simulink model "robotSafeTrajectoryTracking"  (R2024a)
settings: Solver=FixedStepAuto  StartTime=0.0  StopTime=20  FixedStep=0.005  RelTol=1e-3
PostLoadFcn:
  | % load sawyer robot mesh for visualization
  | exampleHelperLoadSawyerMesh()
InitFcn:
  | objectPos = 0.6;
  | refPos = 0.185;
StartFcn:
  | objectPos = 0.6;
model workspace (MAT data in the model file):
  p = [0  0.0291358024691  0  -0.0538271604938  0  0.0247111111111  -0.0818790123457; 0  -0.218518518519  0  0.403703703704  0  -0.185333333333  0.614092592593; 0  0.437037037037  0  -0.807407407407  0  0.370666666667  -1.22818518519; 0  0  0  0  0  0  0; 0  0  0  0  0  0  0; 0  -1.18  0  2.18  0  -1.0008  3.3161]
  q0 = [0; -1.18; 0; 2.18; 0; -1.0008; 3.3161]
  q1 = [0; 0; 0; 0; 0; 0; 0]
  sawyer : robotics.RigidBodyTree (value not decoded)
  tDuration = 3
  tStart = 0.5
undefined symbols (not defined in the file or in its folder): X, Y, Z
libraries: sm_lib x153, nesl_utility x33, robotmaniplib x5, robotcorelib x2
(part 1 of 4)
CloseFcn:
  | clear objectPos refPos
settings Model: Creator=The MathWorks, Inc.  LastModifiedBy=amazon
settings SolverCC: AlgebraicLoopSolver=TrustRegion  MinimalZcImpactIntegration=on
settings DataIOCC: ReturnWorkspaceOutputs=off
settings DebuggingCC: UnconnectedInputMsg=warning  UnconnectedOutputMsg=warning  UnconnectedLineMsg=warning  ArithmeticOperatorsInVariantConditions=warning
settings ModelReferenceCC: EnableRefExpFcnMdlSchedulingChecks=on
settings SFSimCC: SimUseLocalCustomCode=off  CustomCodeUndefinedFunction=UseInterfaceOnly
settings RTWCC: RTWUseLocalCustomCode=off  GPUComputeCapability=3.5  DLArmComputeVersion=19.05
settings DiagnosticsConfigSet: SimMechanicsRigidlyBoundBlock=warning

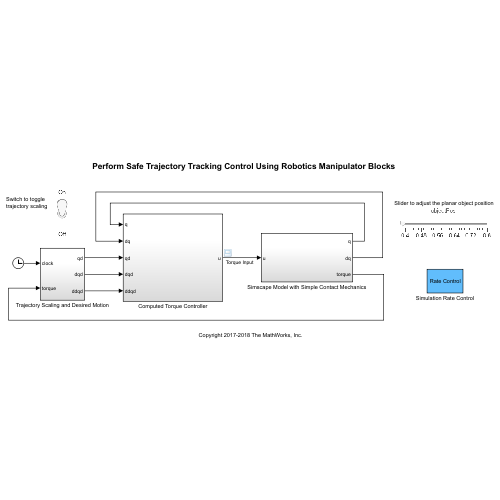
[thumbnail: Simulink's stored preview of the top-level diagram]
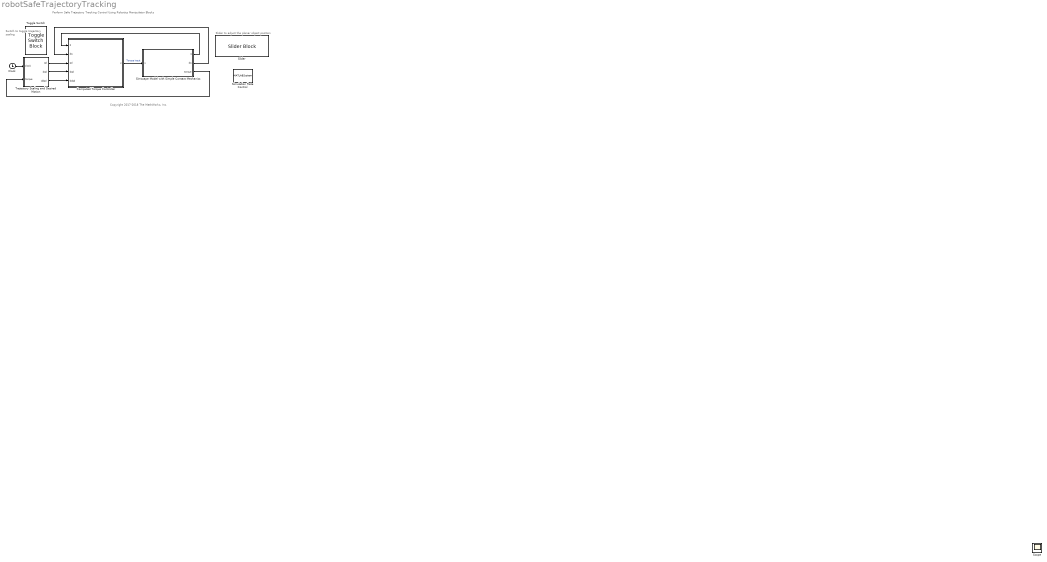
== system robotSafeTrajectoryTracking ==
  note: Perform Safe Trajectory Tracking Control Using Robotics Manipulator Blocks
  note: Switch to toggle
      | trajectory scaling
  note: Copyright 2017-2018 The MathWorks, Inc.
  note: Slider to adjust the planar object position
  Clock : Clock
  Computed Torque Controller : Subsystem
  Simscape Model with Simple Contact Mechanics : Subsystem
  Simulation Rate Control : MATLABSystem  System=ExampleHelperSimulationRateControl  SampleTime=0.005
      mask Type: ExampleHelperSimulationRateControl
      mask Display: disp('Rate Control');
  Slider : SliderBlock  ScaleMin=0.40000000000000002  ScaleMax=0.80000000000000004
  Toggle Switch : ToggleSwitchBlock  LabelPosition=Hide
      settings: Values={{'Off', 'On'}, [0 1]}
  Trajectory Scaling and Desired Motion : Subsystem
  Scope : Scope
  wires:
  Trajectory Scaling and Desired Motion/1(qd) -> Computed Torque Controller/3(qd)
  Trajectory Scaling and Desired Motion/2(dqd) -> Computed Torque Controller/4(dqd)
  Trajectory Scaling and Desired Motion/3(ddqd) -> Computed Torque Controller/5(ddqd)
  Clock/1 -> Trajectory Scaling and Desired Motion/1(clock)
  Simscape Model with Simple Contact Mechanics/1(q) -> Computed Torque Controller/1(q)
  Simscape Model with Simple Contact Mechanics/2(dq) -> Computed Torque Controller/2(dq)
  Simscape Model with Simple Contact Mechanics/3(torque) -> Trajectory Scaling and Desired Motion/2(torque)
  Computed Torque Controller/1(u) -> Simscape Model with Simple Contact Mechanics/1(u)  "Torque Input"

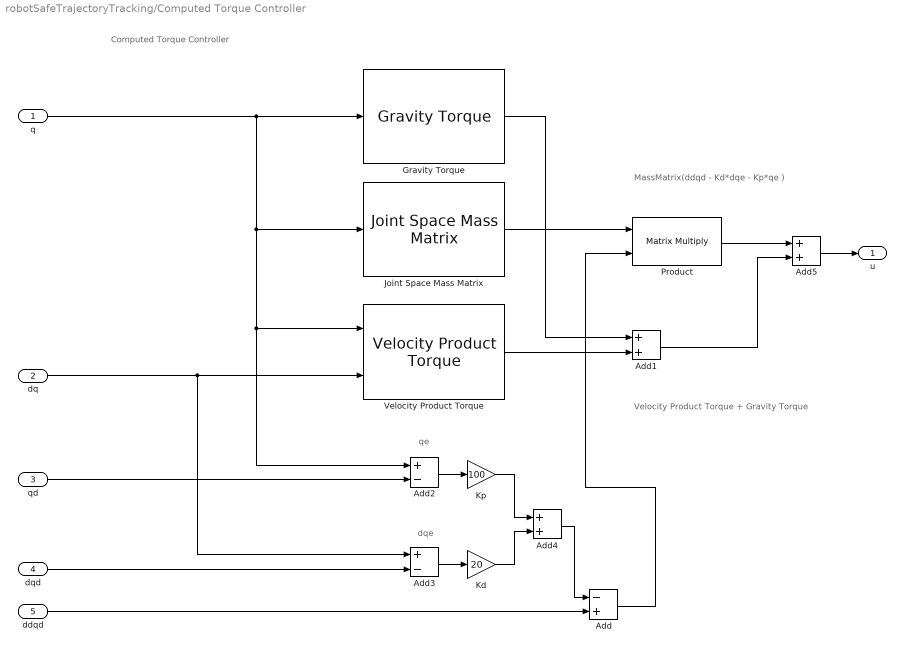
== system robotSafeTrajectoryTracking/Computed Torque Controller ==
  note: qe
  note: dqe
  note: Velocity Product Torque + Gravity Torque
  note: MassMatrix(ddqd - Kd*dqe - Kp*qe )
  note: Computed Torque Controller
  q : Inport
  dq : Inport  Port=2
  qd : Inport  Port=3
  dqd : Inport  Port=4
  ddqd : Inport  Port=5
  Add : Sum  Inputs=-+
  Add1 : Sum
  Add2 : Sum  Inputs=+-
  Add3 : Sum  Inputs=+-
  Add4 : Sum
  Add5 : Sum
  Gravity Torque : robotmaniplib/Gravity Torque  RigidBodyTree=sawyer  SimulateUsing=Interpreted execution
  Joint Space Mass Matrix : robotmaniplib/Joint Space Mass Matrix  RigidBodyTree=sawyer  SimulateUsing=Interpreted execution
  Kd : Gain  Gain=20
  Kp : Gain  Gain=100
  Product : Product  Multiplication=Matrix(*)
  Velocity Product Torque : robotmaniplib/Velocity Product Torque  RigidBodyTree=sawyer  SimulateUsing=Interpreted execution
  u : Outport  VectorParamsAs1DForOutWhenUnconnected=off
  wires:
  Joint Space Mass Matrix/1 -> Product/1
  q/1 -> Gravity Torque/1, Joint Space Mass Matrix/1, Add2/1, Velocity Product Torque/1
  dq/1 -> Velocity Product Torque/2, Add3/1
  Add4/1 -> Add/1
  ddqd/1 -> Add/2
  Add/1 -> Product/2
  qd/1 -> Add2/2
  dqd/1 -> Add3/2
  Add2/1 -> Kp/1
  Add3/1 -> Kd/1
  Kp/1 -> Add4/1
  Kd/1 -> Add4/2
  Add5/1 -> u/1
  Product/1 -> Add5/1
  Add1/1 -> Add5/2
  Gravity Torque/1 -> Add1/1
  Velocity Product Torque/1 -> Add1/2

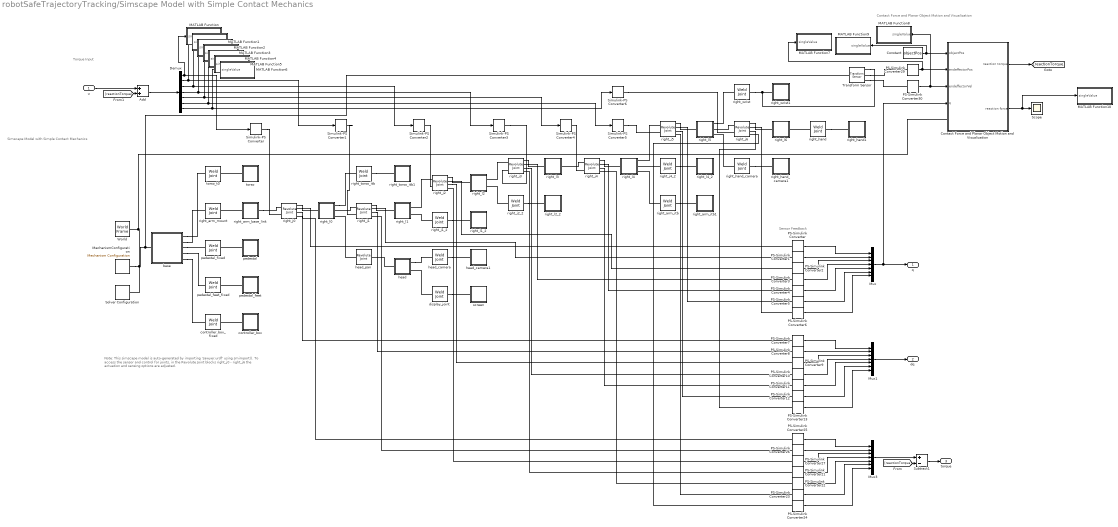
== system robotSafeTrajectoryTracking/Simscape Model with Simple Contact Mechanics ==
  note: Contact Force and Planar Object Motion and Visualization
  note: Sensor Feedback
  note: Torque Input
  note: Simscape Model with Simple Contact Mechanics
  note: Note: This simscape model is auto-generated by importing 'sawyer.urdf' using smimport().
      | To access the sensor and control for joints, in the Revolute Joint blocks right_j0 - right_j6
      | the actuation and sensing options are adjusted.
  u : Inport
  Add : Sum
  Constant : Constant  Value=objectPos
  Contact Force and Planar Object Motion and Visualization : Subsystem
  Demux : Demux  Outputs=7
  MATLAB Function : MATLAB Function  TreatAsAtomicUnit=on
  MATLAB Function1 : MATLAB Function  TreatAsAtomicUnit=on
  MATLAB Function10 : MATLAB Function  TreatAsAtomicUnit=on
  MATLAB Function2 : MATLAB Function  TreatAsAtomicUnit=on
  MATLAB Function3 : MATLAB Function  TreatAsAtomicUnit=on
  MATLAB Function4 : MATLAB Function  TreatAsAtomicUnit=on
  MATLAB Function5 : MATLAB Function  TreatAsAtomicUnit=on
  MATLAB Function6 : MATLAB Function  TreatAsAtomicUnit=on
  MATLAB Function7 : MATLAB Function  TreatAsAtomicUnit=on
  MATLAB Function8 : MATLAB Function  TreatAsAtomicUnit=on
  MATLAB Function9 : MATLAB Function  TreatAsAtomicUnit=on
  MechanismConfiguration : sm_lib/Utilities/Mechanism Configuration  UniformGravity=Constant  GravityVector=[0 0 -9.80665]  GravityVectorUnits=m/s^2  LinearizationDelta=0.001  JointModeTransitionNonlinearIterations=2
  Mux : Mux  Inputs=7
  Mux1 : Mux  Inputs=7
  Mux3 : Mux  Inputs=7
  PS-Simulink Converter{,1..13,21..27,29..30} (23 alike) : nesl_utility/PS-Simulink Converter  PhysicalDomain=network_engine_domain  SubClassName=ps_output  LeftPortType=input  RightPortType=output  PseudoPeriodic=off  Frequencies=[]  VectorFormat=1-D array  Unit=1  AffineConversion=off
  Scope : Scope
  Simulink-PS Converter{,1..6} (7 alike) : nesl_utility/Simulink-PS Converter  PhysicalDomain=network_engine_domain  SubClassName=ps_input  LeftPortType=input  RightPortType=output  PseudoPeriodic=off  Frequencies=[]  NoiseDistribution=none  NoiseParameters=[]  Unit=1  AffineConversion=off  FilteringAndDerivatives=provide  SimscapeFilterOrder=1  InputFilterTimeConstant=0.001  UdotUserProvided=0
  Solver Configuration : nesl_utility/Solver Configuration  PhysicalDomain=network_engine_domain  SubClassName=solver  LeftPortType=input  RightPortType=generic  Tones=[]  Harmonics=[]  SimulateNoise=off  Profile=off  UseLocalSampling=off  EnableSwitchedLinearOptims=on  FrequencyDomain=off  UseCCode=off  RelTol=0.001  AbsTol=1e-06  MinStep=1e-09  ToWorkspace=off  RevertToSquareIcSolve=off  NumHomotopyIterations=100  PhasorMode=off  PhasorModeNumHarmonics=1  ConsistencySolver=NEWTON_FTOL  IndexReductionMethod=DerivativeReplacement  DoDC=off  ResidualTolerance=1e-09  ConsistencyTolSource=GLOBAL  ConsistencyAbsTol=0.001  ConsistencyRelTol=0.001  ConsistencyTolFactor=0.001  UseLocalSolver=off  LocalSolverChoice=NE_BACKWARD_EULER_ADVANCER  ResolveIndetEquations=on  FunctionEvalNumThread=1  LocalSolverSampleTime=0.001  DoFixedCost=off  MaxNonlinIter=3  MaxModeIter=2  ComputeImpulses=off  ImpulseIterations=2  LinearAlgebra=Sparse  LinearAlgebraNumThread=0  EquationFormulation=NE_TIME_EF  DelaysMemoryBudget=1024  AutomaticFiltering=on  FilteringTimeConstant=0.001  PartitionStorageMethod=AS_NEEDED  PartitionMemoryBudget=1024  PartitionMethod=FAST  MultibodyUseLocalSolver=off  MultibodyLocalSolverChoice=ODE1  MultibodyLocalSolverSampleTime=0.001
  Subtract1 : Sum  Inputs=+-
  Transform Sensor : sm_lib/Frames and Transforms/Transform Sensor  MeasurementFrame=World  RotationSequence=XYX  SenseAngle=off  SenseAxis=off  SenseQ=off  SenseR=off  SenseRotationSequence=off  SenseOmegaX=off  SenseOmegaY=off  SenseOmegaZ=off  SenseOmega=off  SenseQDot=off  SenseRDot=off  SenseRotationSequenceDot=off  SenseAlphaX=off  SenseAlphaY=off  SenseAlphaZ=off  SenseAlpha=off  SenseQDDot=off  SenseRDDot=off  SenseX=on  SenseY=off  SenseZ=off  SenseXYZ=off  SenseRad=off  SenseAzim=off  SenseDist=off  SenseInc=off  SenseXDot=on  SenseYDot=off  SenseZDot=off  SenseXYZDot=off  SenseRadDot=off  SenseAzimDot=off  SenseDistDot=off  SenseIncDot=off  SenseXDDot=off  SenseYDDot=off  SenseZDDot=off  SenseXYZDDot=off  SenseRadDDot=off  SenseAzimDDot=off  SenseDistDDot=off  SenseIncDDot=off
  World : sm_lib/Frames and Transforms/World Frame
  base : Subsystem
  controller_box : Subsystem
  controller_box_fixed : sm_lib/Joints/Weld Joint  JointMode=Normal  CompositeWrenchDir=FollowerOnBase  CompositeWrenchFrame=BaseFrame  SenseConstraintForce=off  SenseConstraintTorque=off  SenseTotalForce=off  SenseTotalTorque=off
  display_joint : sm_lib/Joints/Weld Joint  JointMode=Normal  CompositeWrenchDir=FollowerOnBase  CompositeWrenchFrame=BaseFrame  SenseConstraintForce=off  SenseConstraintTorque=off  SenseTotalForce=off  SenseTotalTorque=off
  head : Subsystem
  head_camera : sm_lib/Joints/Weld Joint  JointMode=Normal  CompositeWrenchDir=FollowerOnBase  CompositeWrenchFrame=BaseFrame  SenseConstraintForce=off  SenseConstraintTorque=off  SenseTotalForce=off  SenseTotalTorque=off
  head_camera1 : Subsystem
  head_pan : sm_lib/Joints/Revolute Joint  JointMode=Normal  CompositeWrenchDir=FollowerOnBase  CompositeWrenchFrame=BaseFrame  SenseConstraintForce=off  SenseConstraintTorque=off  SenseTotalForce=off  SenseTotalTorque=off  PositionTargetSpecify=off  PositionTargetPriority=High  PositionTargetValue=0  PositionTargetValueUnits=deg  VelocityTargetSpecify=off  VelocityTargetPriority=High  VelocityTargetValue=0  VelocityTargetValueUnits=deg/s  EquilibriumPosition=0  EquilibriumPositionUnits=deg  SpringStiffness=0  SpringStiffnessUnits=N*m/deg  DampingCoefficient=0  DampingCoefficientUnits=m^2*kg/s/rad  LowerLimitSpecify=off  LowerLimitBound=-90  LowerLimitBoundUnits=deg  LowerLimitStiffness=1e4  LowerLimitStiffnessUnits=N*m/deg  LowerLimitDamping=10  LowerLimitDampingUnits=N*m/(deg/s)  LowerLimitTransitionRegionWidth=0.1  LowerLimitTransitionRegionWidthUnits=deg  UpperLimitSpecify=off  UpperLimitBound=90  UpperLimitBoundUnits=deg  UpperLimitStiffness=1e4  UpperLimitStiffnessUnits=N*m/deg  UpperLimitDamping=10  UpperLimitDampingUnits=N*m/(deg/s)  UpperLimitTransitionRegionWidth=0.1  UpperLimitTransitionRegionWidthUnits=deg  TorqueActuationMode=NoTorque  MotionActuationMode=ComputedMotion  SensePosition=off  SenseVelocity=off  SenseAcceleration=off  SenseTorqueForce=off  SenseLowerLimitTorqueForce=off  SenseUpperLimitTorqueForce=off
  pedestal : Subsystem
  pedestal_feet : Subsystem
  pedestal_feet_fixed : sm_lib/Joints/Weld Joint  JointMode=Normal  CompositeWrenchDir=FollowerOnBase  CompositeWrenchFrame=BaseFrame  SenseConstraintForce=off  SenseConstraintTorque=off  SenseTotalForce=off  SenseTotalTorque=off
  pedestal_fixed : sm_lib/Joints/Weld Joint  JointMode=Normal  CompositeWrenchDir=FollowerOnBase  CompositeWrenchFrame=BaseFrame  SenseConstraintForce=off  SenseConstraintTorque=off  SenseTotalForce=off  SenseTotalTorque=off
  right_arm_base_link : Subsystem
  right_arm_itb : sm_lib/Joints/Weld Joint  JointMode=Normal  CompositeWrenchDir=FollowerOnBase  CompositeWrenchFrame=BaseFrame  SenseConstraintForce=off  SenseConstraintTorque=off  SenseTotalForce=off  SenseTotalTorque=off
  right_arm_itb1 : Subsystem
  right_arm_mount : sm_lib/Joints/Weld Joint  JointMode=Normal  CompositeWrenchDir=FollowerOnBase  CompositeWrenchFrame=BaseFrame  SenseConstraintForce=off  SenseConstraintTorque=off  SenseTotalForce=off  SenseTotalTorque=off
  right_hand : sm_lib/Joints/Weld Joint  JointMode=Normal  CompositeWrenchDir=FollowerOnBase  CompositeWrenchFrame=BaseFrame  SenseConstraintForce=off  SenseConstraintTorque=off  SenseTotalForce=off  SenseTotalTorque=off
  right_hand1 : Subsystem
  right_hand_camera : sm_lib/Joints/Weld Joint  JointMode=Normal  CompositeWrenchDir=FollowerOnBase  CompositeWrenchFrame=BaseFrame  SenseConstraintForce=off  SenseConstraintTorque=off  SenseTotalForce=off  SenseTotalTorque=off
  right_hand_camera1 : Subsystem
  right_j0 : sm_lib/Joints/Revolute Joint  JointMode=Normal  CompositeWrenchDir=FollowerOnBase  CompositeWrenchFrame=BaseFrame  SenseConstraintForce=off  SenseConstraintTorque=off  SenseTotalForce=off  SenseTotalTorque=off  PositionTargetSpecify=on  PositionTargetPriority=High  PositionTargetValue=q0(1)  PositionTargetValueUnits=rad  VelocityTargetSpecify=off  VelocityTargetPriority=High  VelocityTargetValue=0  VelocityTargetValueUnits=deg/s  EquilibriumPosition=0  EquilibriumPositionUnits=deg  SpringStiffness=0  SpringStiffnessUnits=N*m/deg  DampingCoefficient=0  DampingCoefficientUnits=m^2*kg/s/rad  LowerLimitSpecify=off  LowerLimitBound=-90  LowerLimitBoundUnits=deg  LowerLimitStiffness=1e4  LowerLimitStiffnessUnits=N*m/deg  LowerLimitDamping=10  LowerLimitDampingUnits=N*m/(deg/s)  LowerLimitTransitionRegionWidth=0.1  LowerLimitTransitionRegionWidthUnits=deg  UpperLimitSpecify=off  UpperLimitBound=90  UpperLimitBoundUnits=deg  UpperLimitStiffness=1e4  UpperLimitStiffnessUnits=N*m/deg  UpperLimitDamping=10  UpperLimitDampingUnits=N*m/(deg/s)  UpperLimitTransitionRegionWidth=0.1  UpperLimitTransitionRegionWidthUnits=deg  TorqueActuationMode=InputTorque  MotionActuationMode=ComputedMotion  SensePosition=on  SenseVelocity=on  SenseAcceleration=off  SenseTorqueForce=on  SenseLowerLimitTorqueForce=off  SenseUpperLimitTorqueForce=off
  right_j1 : sm_lib/Joints/Revolute Joint  JointMode=Normal  CompositeWrenchDir=FollowerOnBase  CompositeWrenchFrame=BaseFrame  SenseConstraintForce=off  SenseConstraintTorque=off  SenseTotalForce=off  SenseTotalTorque=off  PositionTargetSpecify=on  PositionTargetPriority=High  PositionTargetValue=q0(2)  PositionTargetValueUnits=rad  VelocityTargetSpecify=off  VelocityTargetPriority=High  VelocityTargetValue=0  VelocityTargetValueUnits=deg/s  EquilibriumPosition=0  EquilibriumPositionUnits=deg  SpringStiffness=0  SpringStiffnessUnits=N*m/deg  DampingCoefficient=0  DampingCoefficientUnits=m^2*kg/s/rad  LowerLimitSpecify=off  LowerLimitBound=-90  LowerLimitBoundUnits=deg  LowerLimitStiffness=1e4  LowerLimitStiffnessUnits=N*m/deg  LowerLimitDamping=10  LowerLimitDampingUnits=N*m/(deg/s)  LowerLimitTransitionRegionWidth=0.1  LowerLimitTransitionRegionWidthUnits=deg  UpperLimitSpecify=off  UpperLimitBound=90  UpperLimitBoundUnits=deg  UpperLimitStiffness=1e4  UpperLimitStiffnessUnits=N*m/deg  UpperLimitDamping=10  UpperLimitDampingUnits=N*m/(deg/s)  UpperLimitTransitionRegionWidth=0.1  UpperLimitTransitionRegionWidthUnits=deg  TorqueActuationMode=InputTorque  MotionActuationMode=ComputedMotion  SensePosition=on  SenseVelocity=on  SenseAcceleration=off  SenseTorqueForce=on  SenseLowerLimitTorqueForce=off  SenseUpperLimitTorqueForce=off
  right_j1_2 : sm_lib/Joints/Weld Joint  JointMode=Normal  CompositeWrenchDir=FollowerOnBase  CompositeWrenchFrame=BaseFrame  SenseConstraintForce=off  SenseConstraintTorque=off  SenseTotalForce=off  SenseTotalTorque=off
  right_j2 : sm_lib/Joints/Revolute Joint  JointMode=Normal  CompositeWrenchDir=FollowerOnBase  CompositeWrenchFrame=BaseFrame  SenseConstraintForce=off  SenseConstraintTorque=off  SenseTotalForce=off  SenseTotalTorque=off  PositionTargetSpecify=on  PositionTargetPriority=High  PositionTargetValue=q0(3)  PositionTargetValueUnits=rad  VelocityTargetSpecify=off  VelocityTargetPriority=High  VelocityTargetValue=0  VelocityTargetValueUnits=deg/s  EquilibriumPosition=0  EquilibriumPositionUnits=deg  SpringStiffness=0  SpringStiffnessUnits=N*m/deg  DampingCoefficient=0  DampingCoefficientUnits=m^2*kg/s/rad  LowerLimitSpecify=off  LowerLimitBound=-90  LowerLimitBoundUnits=deg  LowerLimitStiffness=1e4  LowerLimitStiffnessUnits=N*m/deg  LowerLimitDamping=10  LowerLimitDampingUnits=N*m/(deg/s)  LowerLimitTransitionRegionWidth=0.1  LowerLimitTransitionRegionWidthUnits=deg  UpperLimitSpecify=off  UpperLimitBound=90  UpperLimitBoundUnits=deg  UpperLimitStiffness=1e4  UpperLimitStiffnessUnits=N*m/deg  UpperLimitDamping=10  UpperLimitDampingUnits=N*m/(deg/s)  UpperLimitTransitionRegionWidth=0.1  UpperLimitTransitionRegionWidthUnits=deg  TorqueActuationMode=InputTorque  MotionActuationMode=ComputedMotion  SensePosition=on  SenseVelocity=on  SenseAcceleration=off  SenseTorqueForce=on  SenseLowerLimitTorqueForce=off  SenseUpperLimitTorqueForce=off
  right_j2_2 : sm_lib/Joints/Weld Joint  JointMode=Normal  CompositeWrenchDir=FollowerOnBase  CompositeWrenchFrame=BaseFrame  SenseConstraintForce=off  SenseConstraintTorque=off  SenseTotalForce=off  SenseTotalTorque=off
  right_j3 : sm_lib/Joints/Revolute Joint  JointMode=Normal  CompositeWrenchDir=FollowerOnBase  CompositeWrenchFrame=BaseFrame  SenseConstraintForce=off  SenseConstraintTorque=off  SenseTotalForce=off  SenseTotalTorque=off  PositionTargetSpecify=on  PositionTargetPriority=High  PositionTargetValue=q0(4)  PositionTargetValueUnits=rad  VelocityTargetSpecify=off  VelocityTargetPriority=High  VelocityTargetValue=0  VelocityTargetValueUnits=deg/s  EquilibriumPosition=0  EquilibriumPositionUnits=deg  SpringStiffness=0  SpringStiffnessUnits=N*m/deg  DampingCoefficient=0  DampingCoefficientUnits=m^2*kg/s/rad  LowerLimitSpecify=off  LowerLimitBound=-90  LowerLimitBoundUnits=deg  LowerLimitStiffness=1e4  LowerLimitStiffnessUnits=N*m/deg  LowerLimitDamping=10  LowerLimitDampingUnits=N*m/(deg/s)  LowerLimitTransitionRegionWidth=0.1  LowerLimitTransitionRegionWidthUnits=deg  UpperLimitSpecify=off  UpperLimitBound=90  UpperLimitBoundUnits=deg  UpperLimitStiffness=1e4  UpperLimitStiffnessUnits=N*m/deg  UpperLimitDamping=10  UpperLimitDampingUnits=N*m/(deg/s)  UpperLimitTransitionRegionWidth=0.1  UpperLimitTransitionRegionWidthUnits=deg  TorqueActuationMode=InputTorque  MotionActuationMode=ComputedMotion  SensePosition=on  SenseVelocity=on  SenseAcceleration=off  SenseTorqueForce=on  SenseLowerLimitTorqueForce=off  SenseUpperLimitTorqueForce=off
  right_j4 : sm_lib/Joints/Revolute Joint  JointMode=Normal  CompositeWrenchDir=FollowerOnBase  CompositeWrenchFrame=BaseFrame  SenseConstraintForce=off  SenseConstraintTorque=off  SenseTotalForce=off  SenseTotalTorque=off  PositionTargetSpecify=on  PositionTargetPriority=High  PositionTargetValue=q0(5)  PositionTargetValueUnits=rad  VelocityTargetSpecify=off  VelocityTargetPriority=High  VelocityTargetValue=0  VelocityTargetValueUnits=deg/s  EquilibriumPosition=0  EquilibriumPositionUnits=deg  SpringStiffness=0  SpringStiffnessUnits=N*m/deg  DampingCoefficient=0  DampingCoefficientUnits=m^2*kg/s/rad  LowerLimitSpecify=off  LowerLimitBound=-90  LowerLimitBoundUnits=deg  LowerLimitStiffness=1e4  LowerLimitStiffnessUnits=N*m/deg  LowerLimitDamping=10  LowerLimitDampingUnits=N*m/(deg/s)  LowerLimitTransitionRegionWidth=0.1  LowerLimitTransitionRegionWidthUnits=deg  UpperLimitSpecify=off  UpperLimitBound=90  UpperLimitBoundUnits=deg  UpperLimitStiffness=1e4  UpperLimitStiffnessUnits=N*m/deg  UpperLimitDamping=10  UpperLimitDampingUnits=N*m/(deg/s)  UpperLimitTransitionRegionWidth=0.1  UpperLimitTransitionRegionWidthUnits=deg  TorqueActuationMode=InputTorque  MotionActuationMode=ComputedMotion  SensePosition=on  SenseVelocity=on  SenseAcceleration=off  SenseTorqueForce=on  SenseLowerLimitTorqueForce=off  SenseUpperLimitTorqueForce=off
  right_j4_2 : sm_lib/Joints/Weld Joint  JointMode=Normal  CompositeWrenchDir=FollowerOnBase  CompositeWrenchFrame=BaseFrame  SenseConstraintForce=off  SenseConstraintTorque=off  SenseTotalForce=off  SenseTotalTorque=off
  right_j5 : sm_lib/Joints/Revolute Joint  JointMode=Normal  CompositeWrenchDir=FollowerOnBase  CompositeWrenchFrame=BaseFrame  SenseConstraintForce=off  SenseConstraintTorque=off  SenseTotalForce=off  SenseTotalTorque=off  PositionTargetSpecify=on  PositionTargetPriority=High  PositionTargetValue=q0(6)  PositionTargetValueUnits=rad  VelocityTargetSpecify=off  VelocityTargetPriority=High  VelocityTargetValue=0  VelocityTargetValueUnits=deg/s  EquilibriumPosition=0  EquilibriumPositionUnits=deg  SpringStiffness=0  SpringStiffnessUnits=N*m/deg  DampingCoefficient=0  DampingCoefficientUnits=m^2*kg/s/rad  LowerLimitSpecify=off  LowerLimitBound=-90  LowerLimitBoundUnits=deg  LowerLimitStiffness=1e4  LowerLimitStiffnessUnits=N*m/deg  LowerLimitDamping=10  LowerLimitDampingUnits=N*m/(deg/s)  LowerLimitTransitionRegionWidth=0.1  LowerLimitTransitionRegionWidthUnits=deg  UpperLimitSpecify=off  UpperLimitBound=90  UpperLimitBoundUnits=deg  UpperLimitStiffness=1e4  UpperLimitStiffnessUnits=N*m/deg  UpperLimitDamping=10  UpperLimitDampingUnits=N*m/(deg/s)  UpperLimitTransitionRegionWidth=0.1  UpperLimitTransitionRegionWidthUnits=deg  TorqueActuationMode=InputTorque  MotionActuationMode=ComputedMotion  SensePosition=on  SenseVelocity=on  SenseAcceleration=off  SenseTorqueForce=on  SenseLowerLimitTorqueForce=off  SenseUpperLimitTorqueForce=off
  right_j6 : sm_lib/Joints/Revolute Joint  JointMode=Normal  CompositeWrenchDir=FollowerOnBase  CompositeWrenchFrame=BaseFrame  SenseConstraintForce=off  SenseConstraintTorque=off  SenseTotalForce=off  SenseTotalTorque=off  PositionTargetSpecify=on  PositionTargetPriority=High  PositionTargetValue=q0(7)  PositionTargetValueUnits=rad  VelocityTargetSpecify=off  VelocityTargetPriority=High  VelocityTargetValue=0  VelocityTargetValueUnits=deg/s  EquilibriumPosition=0  EquilibriumPositionUnits=deg  SpringStiffness=0  SpringStiffnessUnits=N*m/deg  DampingCoefficient=0  DampingCoefficientUnits=m^2*kg/s/rad  LowerLimitSpecify=off  LowerLimitBound=-90  LowerLimitBoundUnits=deg  LowerLimitStiffness=1e4  LowerLimitStiffnessUnits=N*m/deg  LowerLimitDamping=10  LowerLimitDampingUnits=N*m/(deg/s)  LowerLimitTransitionRegionWidth=0.1  LowerLimitTransitionRegionWidthUnits=deg  UpperLimitSpecify=off  UpperLimitBound=90  UpperLimitBoundUnits=deg  UpperLimitStiffness=1e4  UpperLimitStiffnessUnits=N*m/deg  UpperLimitDamping=10  UpperLimitDampingUnits=N*m/(deg/s)  UpperLimitTransitionRegionWidth=0.1  UpperLimitTransitionRegionWidthUnits=deg  TorqueActuationMode=InputTorque  MotionActuationMode=ComputedMotion  SensePosition=on  SenseVelocity=on  SenseAcceleration=off  SenseTorqueForce=on  SenseLowerLimitTorqueForce=off  SenseUpperLimitTorqueForce=off
  right_l0 : Subsystem
  right_l1 : Subsystem
  right_l1_2 : Subsystem
  right_l2 : Subsystem
  right_l2_2 : Subsystem
  right_l3 : Subsystem
  right_l4 : Subsystem
  right_l4_2 : Subsystem
  right_l5 : Subsystem
  right_l6 : Subsystem
  right_torso_itb : sm_lib/Joints/Weld Joint  JointMode=Normal  CompositeWrenchDir=FollowerOnBase  CompositeWrenchFrame=BaseFrame  SenseConstraintForce=off  SenseConstraintTorque=off  SenseTotalForce=off  SenseTotalTorque=off
  right_torso_itb1 : Subsystem
  right_wrist : sm_lib/Joints/Weld Joint  JointMode=Normal  CompositeWrenchDir=FollowerOnBase  CompositeWrenchFrame=BaseFrame  SenseConstraintForce=off  SenseConstraintTorque=off  SenseTotalForce=off  SenseTotalTorque=off
  right_wrist1 : Subsystem
  screen : Subsystem
  torso : Subsystem
  torso_t0 : sm_lib/Joints/Weld Joint  JointMode=Normal  CompositeWrenchDir=FollowerOnBase  CompositeWrenchFrame=BaseFrame  SenseConstraintForce=off  SenseConstraintTorque=off  SenseTotalForce=off  SenseTotalTorque=off
  q : Outport  VectorParamsAs1DForOutWhenUnconnected=off
  dq : Outport  Port=2  VectorParamsAs1DForOutWhenUnconnected=off
  torque : Outport  Port=3  VectorParamsAs1DForOutWhenUnconnected=off
  wires:
  Demux/7 -> MATLAB Function6/1(singleValue), Simulink-PS Converter6/1
  Demux/6 -> MATLAB Function5/1(singleValue), Simulink-PS Converter5/1
  Demux/2 -> MATLAB Function1/1(singleValue), Simulink-PS Converter1/1
  Demux/1 -> MATLAB Function/1(singleValue), Simulink-PS Converter/1
  Demux/3 -> MATLAB Function2/1(singleValue), Simulink-PS Converter2/1
  Demux/5 -> MATLAB Function4/1(singleValue), Simulink-PS Converter4/1
  Demux/4 -> MATLAB Function3/1(singleValue), Simulink-PS Converter3/1
  PS-Simulink Converter10/1 -> Mux1/4
  PS-Simulink Converter5/1 -> Mux/6
  PS-Simulink Converter8/1 -> Mux1/2
  PS-Simulink Converter13/1 -> Mux1/7
  PS-Simulink Converter3/1 -> Mux/4
  PS-Simulink Converter26/1 -> Mux3/2
  PS-Simulink Converter22/1 -> Mux3/5
  PS-Simulink Converter12/1 -> Mux1/6
  PS-Simulink Converter27/1 -> Mux3/3
  Mux/1 -> Contact Force and Planar Object Motion and Visualization/4(q), q/1
  PS-Simulink Converter24/1 -> Mux3/7
  Mux1/1 -> dq/1
  PS-Simulink Converter4/1 -> Mux/5
  PS-Simulink Converter6/1 -> Mux/7
  PS-Simulink Converter7/1 -> Mux1/1
  PS-Simulink Converter11/1 -> Mux1/5
  PS-Simulink Converter23/1 -> Mux3/6
  PS-Simulink Converter25/1 -> Mux3/1
  PS-Simulink Converter/1 -> Mux/1
  PS-Simulink Converter21/1 -> Mux3/4
  PS-Simulink Converter2/1 -> Mux/3
  PS-Simulink Converter9/1 -> Mux1/3
  PS-Simulink Converter1/1 -> Mux/2
  Mux3/1 -> Subtract1/1
  [reactionTorque] -> Subtract1/2
  Subtract1/1 -> torque/1
  u/1 -> Add/1
  Add/1 -> Demux/1
  [reactionTorque] -> Add/2
  Constant/1 -> MATLAB Function9/1(singleValue), Contact Force and Planar Object Motion and Visualization/1(objectPos)
  PS-Simulink Converter30/1 -> MATLAB Function8/1(singleValue), Contact Force and Planar Object Motion and Visualization/3(endeffectorVel)
  Contact Force and Planar Object Motion and Visualization/1(reaction torque) -> [reactionTorque]
  Contact Force and Planar Object Motion and Visualization/2(reaction force) -> MATLAB Function10/1(singleValue), Scope/1
  PS-Simulink Converter29/1 -> MATLAB Function7/1(singleValue), Contact Force and Planar Object Motion and Visualization/2(endeffectorPos)
  connections:
  right_j4_2/RConn1 -- right_l4_2/LConn1
  right_j6/RConn1 -- right_l6/LConn1
  base/RConn4 -- pedestal_feet_fixed/LConn1
  right_arm_base_link/LConn1 -- right_arm_mount/RConn1
  right_wrist/RConn1 -- Transform Sensor/RConn1 -- right_wrist1/LConn1
  right_j4_2/LConn1 -- right_l4/RConn2
  pedestal/LConn1 -- pedestal_fixed/RConn1
  head_pan/LConn1 -- right_l0/RConn3
  head_camera/RConn1 -- head_camera1/LConn1
  right_j1_2/RConn1 -- right_l1_2/LConn1
  right_torso_itb/RConn1 -- right_torso_itb1/LConn1
  right_hand/LConn1 -- right_l6/RConn1
  right_arm_base_link/RConn1 -- right_j0/LConn1
  right_hand/RConn1 -- right_hand1/LConn1
  right_arm_itb/LConn1 -- right_l4/RConn3
  right_l0/RConn1 -- right_torso_itb/LConn1
  right_j1_2/LConn1 -- right_l1/RConn2
  right_j3/RConn1 -- right_l3/LConn1
  base/RConn2 -- right_arm_mount/LConn1
  head/LConn1 -- head_pan/RConn1
  right_j4/LConn1 -- right_l3/RConn1
  base/RConn1 -- torso_t0/LConn1
  right_j2_2/RConn1 -- right_l2_2/LConn1
  right_j1/RConn1 -- right_l1/LConn1
  base/RConn5 -- controller_box_fixed/LConn1
  right_hand_camera/LConn1 -- right_l5/RConn3
  right_l5/RConn1 -- right_wrist/LConn1
  pedestal_feet/LConn1 -- pedestal_feet_fixed/RConn1
  right_j1/LConn1 -- right_l0/RConn2
  display_joint/LConn1 -- head/RConn2
  right_j6/LConn1 -- right_l5/RConn2
  base/RConn3 -- pedestal_fixed/LConn1
  display_joint/RConn1 -- screen/LConn1
  right_j2_2/LConn1 -- right_l2/RConn2
  right_j5/LConn1 -- right_l4/RConn1
  right_arm_itb/RConn1 -- right_arm_itb1/LConn1
  right_j0/RConn1 -- right_l0/LConn1
  torso/LConn1 -- torso_t0/RConn1
  right_j5/RConn1 -- right_l5/LConn1
  right_hand_camera/RConn1 -- right_hand_camera1/LConn1
  right_j2/LConn1 -- right_l1/RConn1
  controller_box/LConn1 -- controller_box_fixed/RConn1
  head/RConn1 -- head_camera/LConn1
  right_j2/RConn1 -- right_l2/LConn1
  right_j4/RConn1 -- right_l4/LConn1
  right_j3/LConn1 -- right_l2/RConn1
  Simulink-PS Converter/RConn1 -- right_j0/LConn2
  Simulink-PS Converter1/RConn1 -- right_j1/LConn2
  Simulink-PS Converter2/RConn1 -- right_j2/LConn2
  Simulink-PS Converter3/RConn1 -- right_j3/LConn2
  Simulink-PS Converter4/RConn1 -- right_j4/LConn2
  Simulink-PS Converter5/RConn1 -- right_j5/LConn2
  Simulink-PS Converter6/RConn1 -- right_j6/LConn2
  right_j0/RConn2 -- PS-Simulink Converter/LConn1
  right_j1/RConn2 -- PS-Simulink Converter1/LConn1
  right_j2/RConn2 -- PS-Simulink Converter2/LConn1
  right_j3/RConn2 -- PS-Simulink Converter3/LConn1
  right_j4/RConn2 -- PS-Simulink Converter4/LConn1
  right_j5/RConn2 -- PS-Simulink Converter5/LConn1
  right_j6/RConn2 -- PS-Simulink Converter6/LConn1
  right_j0/RConn3 -- PS-Simulink Converter7/LConn1
  right_j1/RConn3 -- PS-Simulink Converter8/LConn1
  right_j2/RConn3 -- PS-Simulink Converter9/LConn1
  right_j3/RConn3 -- PS-Simulink Converter10/LConn1
  right_j4/RConn3 -- PS-Simulink Converter11/LConn1
  right_j5/RConn3 -- PS-Simulink Converter12/LConn1
  right_j6/RConn3 -- PS-Simulink Converter13/LConn1
  PS-Simulink Converter25/LConn1 -- right_j0/RConn4
  PS-Simulink Converter26/LConn1 -- right_j1/RConn4
  PS-Simulink Converter27/LConn1 -- right_j2/RConn4
  PS-Simulink Converter21/LConn1 -- right_j3/RConn4
  PS-Simulink Converter22/LConn1 -- right_j4/RConn4
  right_j5/RConn4 -- PS-Simulink Converter23/LConn1
  PS-Simulink Converter24/LConn1 -- right_j6/RConn4
  base/LConn1 -- MechanismConfiguration/RConn1 -- Contact Force and Planar Object Motion and Visualization/LConn1 -- World/RConn1 -- Solver Configuration/RConn1 -- Transform Sensor/LConn1
  Transform Sensor/RConn2 -- PS-Simulink Converter29/LConn1
  Transform Sensor/RConn3 -- PS-Simulink Converter30/LConn1

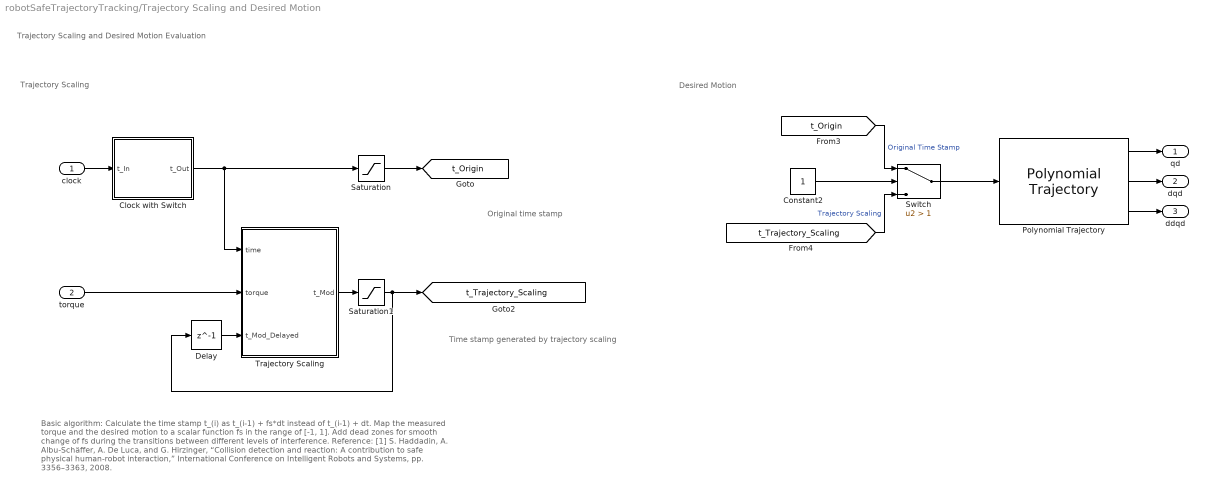
== system robotSafeTrajectoryTracking/Trajectory Scaling and Desired Motion ==
  note: Trajectory Scaling
  note: Desired Motion
  note: Time stamp generated by trajectory scaling
  note: Original time stamp
  note: Trajectory Scaling and Desired Motion Evaluation
  note: Basic algorithm:
      | Calculate the time stamp t_(i) as t_(i-1) + fs*dt instead of t_(i-1) + dt.
      | Map the measured torque and the desired motion to a scalar function fs in the range of [-1, 1].
      | Add dead zones for smooth change of fs during the transitions between different levels of interference.
      |
      | Reference:
      | [1] S. Haddadin, A. Albu-Schäffer, A. De Luca, and G. Hirzinger, “Collision detection and reaction: A contribution to safe physical
      | human-robot interaction,” International Conference on Intelligent Robots and Systems, pp. 3356–3363, 2008.
  clock : Inport
  torque : Inport  Port=2
  Clock with Switch : Subsystem
  Constant2 : Constant
  Delay : Delay  DelayLength=1
  Polynomial Trajectory : robotcorelib/Polynomial Trajectory  WaypointSource=Internal  Waypoints=[q0 q1]  TimePoints=[0 tDuration]  TimeInterval=[ 1, 4 ]  Method=Quintic Polynomial  ParameterSource=Internal  VelocityBoundaryCondition=zeros(numel(q0),2)  AccelerationBoundaryCondition=zeros(numel(q0),2)  SimulateUsing=Interpreted execution
  Saturation : Saturate  UpperLimit=tDuration  LowerLimit=0
  Saturation1 : Saturate  UpperLimit=tDuration  LowerLimit=0
  Switch : Switch  Criteria=u2 > Threshold  Threshold=1  SaturateOnIntegerOverflow=off  InputSameDT=off
  Trajectory Scaling : Subsystem
  qd : Outport  VectorParamsAs1DForOutWhenUnconnected=off
  dqd : Outport  Port=2  VectorParamsAs1DForOutWhenUnconnected=off
  ddqd : Outport  Port=3  VectorParamsAs1DForOutWhenUnconnected=off
  tag scope: t_Origin=global, t_Trajectory_Scaling=global
  wires:
  Trajectory Scaling/1(t_Mod) -> Saturation1/1
  [t_Trajectory_Scaling] -> Switch/3  "Trajectory Scaling"
  Constant2/1 -> Switch/2
  Polynomial Trajectory/1 -> qd/1
  Clock with Switch/1(t_Out) -> Trajectory Scaling/1(time), Saturation/1
  Saturation/1 -> [t_Origin]
  Switch/1 -> Polynomial Trajectory/1
  [t_Origin] -> Switch/1  "Original Time Stamp"
  Saturation1/1 -> Delay/1, [t_Trajectory_Scaling]
  Polynomial Trajectory/3 -> ddqd/1
  Polynomial Trajectory/2 -> dqd/1
  clock/1 -> Clock with Switch/1(t_In)
  torque/1 -> Trajectory Scaling/2(torque)
  Delay/1 -> Trajectory Scaling/3("t_Mod_Delayed ")

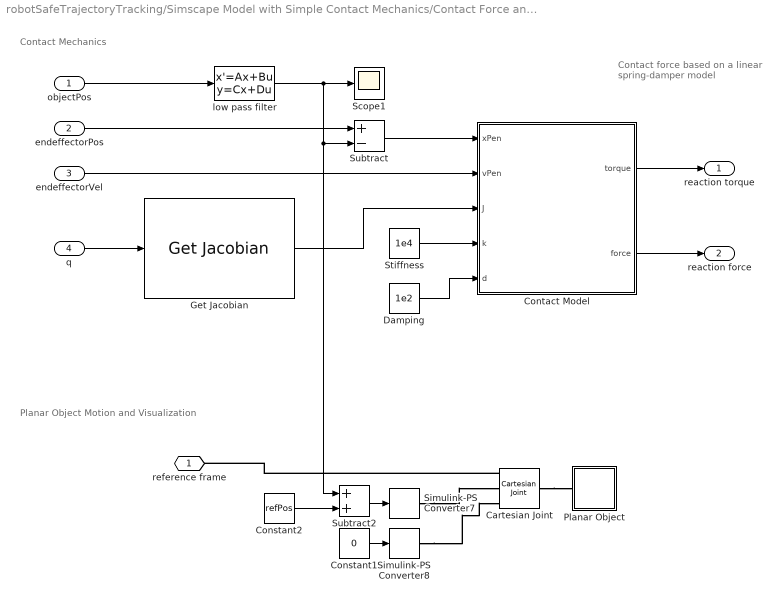
== system robotSafeTrajectoryTracking/Simscape Model with Simple Contact Mechanics/Contact Force and Planar Object Motion and Visualization ==
  note: Planar Object Motion and Visualization
  note: Contact Mechanics
  note: Contact force based on a linear
      | spring-damper model
  objectPos : Inport
  endeffectorPos : Inport  Port=2
  endeffectorVel : Inport  Port=3
  q : Inport  Port=4
  Cartesian Joint : sm_lib/Joints/Cartesian Joint  JointMode=Normal  CompositeWrenchDir=FollowerOnBase  CompositeWrenchFrame=BaseFrame  SenseConstraintForce=off  SenseConstraintTorque=off  SenseTotalForce=off  SenseTotalTorque=off  PxPositionTargetSpecify=on  PxPositionTargetPriority=High  PxPositionTargetValue=0.6+0.19  PxPositionTargetValueUnits=m  PxVelocityTargetSpecify=off  PxVelocityTargetPriority=High  PxVelocityTargetValue=0  PxVelocityTargetValueUnits=m/s  PxEquilibriumPosition=0  PxEquilibriumPositionUnits=m  PxSpringStiffness=0  PxSpringStiffnessUnits=N/m  PxDampingCoefficient=0  PxDampingCoefficientUnits=N/(m/s)  PxLowerLimitSpecify=off  PxLowerLimitBound=-1  PxLowerLimitBoundUnits=m  PxLowerLimitStiffness=1e6  PxLowerLimitStiffnessUnits=N/m  PxLowerLimitDamping=1e3  PxLowerLimitDampingUnits=N/(m/s)  PxLowerLimitTransitionRegionWidth=1e-4  PxLowerLimitTransitionRegionWidthUnits=m  PxUpperLimitSpecify=off  PxUpperLimitBound=1  PxUpperLimitBoundUnits=m  PxUpperLimitStiffness=1e6  PxUpperLimitStiffnessUnits=N/m  PxUpperLimitDamping=1e3  PxUpperLimitDampingUnits=N/(m/s)  PxUpperLimitTransitionRegionWidth=1e-4  PxUpperLimitTransitionRegionWidthUnits=m  PxTorqueActuationMode=ComputedTorque  PxMotionActuationMode=InputMotion  PxSensePosition=off  PxSenseVelocity=off  PxSenseAcceleration=off  PxSenseTorqueForce=off  PxSenseLowerLimitTorqueForce=off  PxSenseUpperLimitTorqueForce=off  PyPositionTargetSpecify=off  PyPositionTargetPriority=High  PyPositionTargetValue=0  PyPositionTargetValueUnits=m  PyVelocityTargetSpecify=off  PyVelocityTargetPriority=High  PyVelocityTargetValue=0  PyVelocityTargetValueUnits=m/s  PyEquilibriumPosition=0  PyEquilibriumPositionUnits=m  PySpringStiffness=0  PySpringStiffnessUnits=N/m  PyDampingCoefficient=0  PyDampingCoefficientUnits=N/(m/s)  PyLowerLimitSpecify=off  PyLowerLimitBound=-1  PyLowerLimitBoundUnits=m  PyLowerLimitStiffness=1e6  PyLowerLimitStiffnessUnits=N/m  PyLowerLimitDamping=1e3  PyLowerLimitDampingUnits=N/(m/s)  PyLowerLimitTransitionRegionWidth=1e-4  PyLowerLimitTransitionRegionWidthUnits=m  PyUpperLimitSpecify=off  PyUpperLimitBound=1  PyUpperLimitBoundUnits=m  PyUpperLimitStiffness=1e6  PyUpperLimitStiffnessUnits=N/m  PyUpperLimitDamping=1e3  PyUpperLimitDampingUnits=N/(m/s)  PyUpperLimitTransitionRegionWidth=1e-4  PyUpperLimitTransitionRegionWidthUnits=m  PyTorqueActuationMode=NoTorque  PyMotionActuationMode=ComputedMotion  PySensePosition=off  PySenseVelocity=off  PySenseAcceleration=off  PySenseTorqueForce=off  PySenseLowerLimitTorqueForce=off  PySenseUpperLimitTorqueForce=off  PzPositionTargetSpecify=off  PzPositionTargetPriority=High  PzPositionTargetValue=0  PzPositionTargetValueUnits=m  PzVelocityTargetSpecify=off  PzVelocityTargetPriority=High  PzVelocityTargetValue=0  PzVelocityTargetValueUnits=m/s  PzEquilibriumPosition=0  PzEquilibriumPositionUnits=m  PzSpringStiffness=0  PzSpringStiffnessUnits=N/m  PzDampingCoefficient=0  PzDampingCoefficientUnits=N/(m/s)  PzLowerLimitSpecify=off  PzLowerLimitBound=-1  PzLowerLimitBoundUnits=m  PzLowerLimitStiffness=1e6  PzLowerLimitStiffnessUnits=N/m  PzLowerLimitDamping=1e3  PzLowerLimitDampingUnits=N/(m/s)  PzLowerLimitTransitionRegionWidth=1e-4  PzLowerLimitTransitionRegionWidthUnits=m  PzUpperLimitSpecify=off  PzUpperLimitBound=1  PzUpperLimitBoundUnits=m  PzUpperLimitStiffness=1e6  PzUpperLimitStiffnessUnits=N/m  PzUpperLimitDamping=1e3  PzUpperLimitDampingUnits=N/(m/s)  PzUpperLimitTransitionRegionWidth=1e-4  PzUpperLimitTransitionRegionWidthUnits=m  PzTorqueActuationMode=ComputedTorque  PzMotionActuationMode=InputMotion  PzSensePosition=off  PzSenseVelocity=off  PzSenseAcceleration=off  PzSenseTorqueForce=off  PzSenseLowerLimitTorqueForce=off  PzSenseUpperLimitTorqueForce=off
  Constant1 : Constant  Value=0
  Constant2 : Constant  Value=refPos
  Contact Model : MATLAB Function  TreatAsAtomicUnit=on
  Damping : Constant  Value=1e2
  Get Jacobian : robotmaniplib/Get Jacobian  RigidBodyTree=sawyer  EndEffector=right_wrist  SimulateUsing=Interpreted execution
  Planar Object : Subsystem
  Scope1 : Scope
  Simulink-PS Converter7 : nesl_utility/Simulink-PS Converter  PhysicalDomain=network_engine_domain  SubClassName=ps_input  LeftPortType=input  RightPortType=output  PseudoPeriodic=off  Frequencies=[]  NoiseDistribution=none  NoiseParameters=[]  Unit=1  AffineConversion=off  FilteringAndDerivatives=filter  SimscapeFilterOrder=2  InputFilterTimeConstant=1e-2  UdotUserProvided=0
  Simulink-PS Converter8 : nesl_utility/Simulink-PS Converter  PhysicalDomain=network_engine_domain  SubClassName=ps_input  LeftPortType=input  RightPortType=output  PseudoPeriodic=off  Frequencies=[]  NoiseDistribution=none  NoiseParameters=[]  Unit=1  AffineConversion=off  FilteringAndDerivatives=provide  SimscapeFilterOrder=2  InputFilterTimeConstant=0.001  UdotUserProvided=0
  Stiffness : Constant  Value=1e4
  Subtract : Sum  Inputs=+-
  Subtract2 : Sum
  low pass filter : StateSpace  A=-10  B=10  D=0  InitialCondition=objectPos
  reference frame : PMIOPort  Side=Left
  reaction torque : Outport  VectorParamsAs1DForOutWhenUnconnected=off
  reaction force : Outport  Port=2  VectorParamsAs1DForOutWhenUnconnected=off
  wires:
  low pass filter/1 -> Scope1/1, Subtract2/1, Subtract/2
  Subtract2/1 -> Simulink-PS Converter7/1
  Get Jacobian/1 -> Contact Model/3(J)
  Constant2/1 -> Subtract2/2
  Contact Model/1(torque) -> reaction torque/1
  Constant1/1 -> Simulink-PS Converter8/1
  Contact Model/2(force) -> reaction force/1
  objectPos/1 -> low pass filter/1
  endeffectorPos/1 -> Subtract/1
  q/1 -> Get Jacobian/1
  Stiffness/1 -> Contact Model/4(k)
  Damping/1 -> Contact Model/5(d)
  Subtract/1 -> Contact Model/1(xPen)
  endeffectorVel/1 -> Contact Model/2(vPen)
  connections:
  Simulink-PS Converter8/RConn1 -- Cartesian Joint/LConn3
  Cartesian Joint/LConn1 -- reference frame/RConn1
  Cartesian Joint/RConn1 -- Planar Object/LConn1
  Simulink-PS Converter7/RConn1 -- Cartesian Joint/LConn2

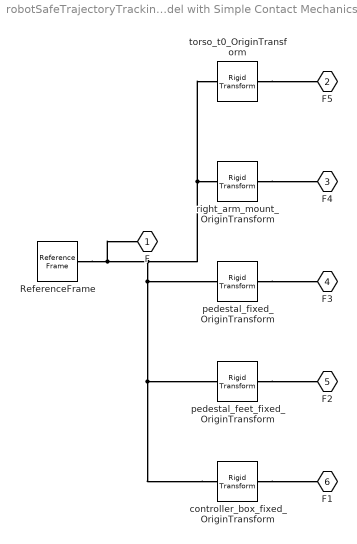
== system robotSafeTrajectoryTracking/Simscape Model with Simple Contact Mechanics/base ==
  ReferenceFrame : sm_lib/Frames and Transforms/Reference Frame
  controller_box_fixed_OriginTransform : sm_lib/Frames and Transforms/Rigid Transform  RotationMethod=RotationSequence  FollAlignAxisA=+X  BaseAlignAxisA=+Y  FollAlignAxisB=+Y  BaseAlignAxisB=+Z  RotationStandardAxis=+Z  RotationAngle=0.0  RotationAngleUnits=deg  RotationArbitraryAxis=[0 0 1]  RotationSequenceAxes=BaseAxes  RotationSequence=XYZ  RotationSequenceAngles=[0, 0, 0]  RotationSequenceAnglesUnits=rad  RotationMatrix=[1 0 0; 0 1 0; 0 0 1]  Quaternion=[1 0 0 0]  TranslationMethod=Cartesian  TranslationCartesianOffset=[0, 0, 0]  TranslationCartesianOffsetUnits=m  TranslationStandardAxis=+Z  TranslationStandardOffset=0  TranslationStandardOffsetUnits=m  TranslationROffset=0  TranslationROffsetUnits=m  TranslationThetaOffset=0  TranslationThetaOffsetUnits=deg  TranslationZOffset=0  TranslationZOffsetUnits=m
  pedestal_feet_fixed_OriginTransform : sm_lib/Frames and Transforms/Rigid Transform  RotationMethod=RotationSequence  FollAlignAxisA=+X  BaseAlignAxisA=+Y  FollAlignAxisB=+Y  BaseAlignAxisB=+Z  RotationStandardAxis=+Z  RotationAngle=0.0  RotationAngleUnits=deg  RotationArbitraryAxis=[0 0 1]  RotationSequenceAxes=BaseAxes  RotationSequence=XYZ  RotationSequenceAngles=[0, 0, 0]  RotationSequenceAnglesUnits=rad  RotationMatrix=[1 0 0; 0 1 0; 0 0 1]  Quaternion=[1 0 0 0]  TranslationMethod=Cartesian  TranslationCartesianOffset=[0, 0, 0]  TranslationCartesianOffsetUnits=m  TranslationStandardAxis=+Z  TranslationStandardOffset=0  TranslationStandardOffsetUnits=m  TranslationROffset=0  TranslationROffsetUnits=m  TranslationThetaOffset=0  TranslationThetaOffsetUnits=deg  TranslationZOffset=0  TranslationZOffsetUnits=m
  pedestal_fixed_OriginTransform : sm_lib/Frames and Transforms/Rigid Transform  RotationMethod=RotationSequence  FollAlignAxisA=+X  BaseAlignAxisA=+Y  FollAlignAxisB=+Y  BaseAlignAxisB=+Z  RotationStandardAxis=+Z  RotationAngle=0.0  RotationAngleUnits=deg  RotationArbitraryAxis=[0 0 1]  RotationSequenceAxes=BaseAxes  RotationSequence=XYZ  RotationSequenceAngles=[0, 0, 0]  RotationSequenceAnglesUnits=rad  RotationMatrix=[1 0 0; 0 1 0; 0 0 1]  Quaternion=[1 0 0 0]  TranslationMethod=Cartesian  TranslationCartesianOffset=[0, 0, 0]  TranslationCartesianOffsetUnits=m  TranslationStandardAxis=+Z  TranslationStandardOffset=0  TranslationStandardOffsetUnits=m  TranslationROffset=0  TranslationROffsetUnits=m  TranslationThetaOffset=0  TranslationThetaOffsetUnits=deg  TranslationZOffset=0  TranslationZOffsetUnits=m
  right_arm_mount_OriginTransform : sm_lib/Frames and Transforms/Rigid Transform  RotationMethod=RotationSequence  FollAlignAxisA=+X  BaseAlignAxisA=+Y  FollAlignAxisB=+Y  BaseAlignAxisB=+Z  RotationStandardAxis=+Z  RotationAngle=0.0  RotationAngleUnits=deg  RotationArbitraryAxis=[0 0 1]  RotationSequenceAxes=BaseAxes  RotationSequence=XYZ  RotationSequenceAngles=[0, 0, 0]  RotationSequenceAnglesUnits=rad  RotationMatrix=[1 0 0; 0 1 0; 0 0 1]  Quaternion=[1 0 0 0]  TranslationMethod=Cartesian  TranslationCartesianOffset=[0, 0, 0]  TranslationCartesianOffsetUnits=m  TranslationStandardAxis=+Z  TranslationStandardOffset=0  TranslationStandardOffsetUnits=m  TranslationROffset=0  TranslationROffsetUnits=m  TranslationThetaOffset=0  TranslationThetaOffsetUnits=deg  TranslationZOffset=0  TranslationZOffsetUnits=m
  torso_t0_OriginTransform : sm_lib/Frames and Transforms/Rigid Transform  RotationMethod=RotationSequence  FollAlignAxisA=+X  BaseAlignAxisA=+Y  FollAlignAxisB=+Y  BaseAlignAxisB=+Z  RotationStandardAxis=+Z  RotationAngle=0.0  RotationAngleUnits=deg  RotationArbitraryAxis=[0 0 1]  RotationSequenceAxes=BaseAxes  RotationSequence=XYZ  RotationSequenceAngles=[0, 0, 0]  RotationSequenceAnglesUnits=rad  RotationMatrix=[1 0 0; 0 1 0; 0 0 1]  Quaternion=[1 0 0 0]  TranslationMethod=Cartesian  TranslationCartesianOffset=[0, 0, 0]  TranslationCartesianOffsetUnits=m  TranslationStandardAxis=+Z  TranslationStandardOffset=0  TranslationStandardOffsetUnits=m  TranslationROffset=0  TranslationROffsetUnits=m  TranslationThetaOffset=0  TranslationThetaOffsetUnits=deg  TranslationZOffset=0  TranslationZOffsetUnits=m
  F : PMIOPort  Side=Left
  F5 : PMIOPort  Port=2  Side=Right
  F4 : PMIOPort  Port=3  Side=Right
  F3 : PMIOPort  Port=4  Side=Right
  F2 : PMIOPort  Port=5  Side=Right
  F1 : PMIOPort  Port=6  Side=Right
  connections:
  controller_box_fixed_OriginTransform/LConn1 -- right_arm_mount_OriginTransform/LConn1 -- torso_t0_OriginTransform/LConn1 -- ReferenceFrame/RConn1 -- F/RConn1 -- pedestal_fixed_OriginTransform/LConn1 -- pedestal_feet_fixed_OriginTransform/LConn1
  controller_box_fixed_OriginTransform/RConn1 -- F1/RConn1
  pedestal_feet_fixed_OriginTransform/RConn1 -- F2/RConn1
  pedestal_fixed_OriginTransform/RConn1 -- F3/RConn1
  right_arm_mount_OriginTransform/RConn1 -- F4/RConn1
  torso_t0_OriginTransform/RConn1 -- F5/RConn1

== system robotSafeTrajectoryTracking/Simscape Model with Simple Contact Mechanics/controller_box ==
  ReferenceFrame : sm_lib/Frames and Transforms/Reference Frame
  F : PMIOPort  Side=Left
  connections:
  ReferenceFrame/RConn1 -- F/RConn1
